simulink library "Condensing_Boiler_CONF"  (R2013b)
settings: Solver=ode45  StartTime=0.0  StopTime=10.0  RelTol=1e-3
libraries: carnot x1
settings Model: Creator=lena.frank  LastModifiedBy=drhf

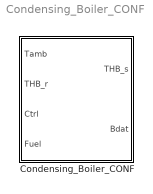
== system Condensing_Boiler_CONF ==
  Condensing_Boiler_CONF : Subsystem  mask(Configurated Condensing Boiler){parameterfile=DefaultCondensingBoiler, tini=20}
      mask prompts: parameterfile "Parameter set"; tini "Inital temperature in °C"
      mask help:
      | Multinode one-dimensional model of a boiler. Condensing effects are taken in account by an efficiency lookup table.
      | This block uses predefined parameter sets.
      mask init:
      | B = CarnotCallbacks_CondensingBoilerConf(parameterfile);
      | relQdotMin = B.QdotMin/B.Qdotnom;
      mask Help: web(fullfile(path_carnot('help'),'Condensing_Boiler_CONF.html'),'-helpbrowser')
      mask TypeOptions parameterfile: DefaultCondensingBoiler | Vitodens_200_13kW | Vitodens_200_19kW | Vitodens_200_26kW | Vitodens_200_35kW
      mask Display:
      | % user defined picture file
      | picfile = fullfile(path_carnot('intlibsl'), ...
      |         'Source','Boiler','Condensing_Boiler_CONF','parameter_set', ...
      |         'Condensing_Boiler_CONF.jpg');
      | 
      | pic = false;
      | if ~BlockIsInCarnotLibrary    % if not located in library any more
      |     if exist(picfile,'file') % show internal picture if defined
      |         image(imread(picfile), [0.2, 0, 0.6, 1])
      |         set_param(gcb, 'BackgroundColor', 'White')
      |         pic = true;
      |     end
      | end
      | if ~pic    % show public picture
      |     set_param(gcb, 'BackgroundColor', 'Red')
      |     plot(0,0,1,1,[10,90,90,10,10]/100,[10,10,20,20,10]/100,[80,80,20,20]/100, ...
      |         [20,90,90,20]/100,[20,70,70,20]/100,[24,24,30,30]/100,[32,30,28]/100, ...
      |         [30,40,30]/100,[43,40,38]/100,[30,40,30]/100,[53,50,47]/100, ...
      |         [30,40,30]/100,[63,60,57]/100,[30,40,30]/100, ...
      |         [35,32,30,29,31,36,39,40,37,35]/100,[75,69,65,58,50,49,53,59,68,75]/100, ...
      |         [57,54,51,51,53,58,62,62,59,57]/100,[76,71,67,58,49,48,54,60,69,76]/100)
      | end
      | 
      | % Show port labels: same as port labels in the subsystem,
      | % but display with a picture covers the text. Have to reprint it.
      | port_label('input',1,'Tamb')
      | port_label('input',2,'THB_r')
      | port_label('input',3,'Ctrl')
      | port_label('input',4,'Fuel')
      | port_label('output',1,'THB_s')
      | port_label('output',2,'Bdat')

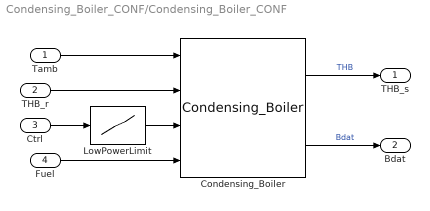
== system Condensing_Boiler_CONF/Condensing_Boiler_CONF ==
  Tamb : Inport
  THB_r : Inport  Port=2
  Ctrl : Inport  Port=3
  Fuel : Inport  Port=4
  Condensing_Boiler : carnot/Source/Boiler/Condensing_Boiler  Pnom=B.Qdotnom  U=B.HeatLoss  vol=B.Volume  electricPower=B.ElectricPower  relativeQdot=B.TableRelativePower  whichTforEfficiency=mean of inlet and outlet temperature  temperatures=B.TableTemperatures  efficiency=B.TableData  lin=B.dplin  qua=B.dpqua  Tini=tini  nodes=B.Nodes
  LowPowerLimit : Lookup  InputValues=[-1, relQdotMin-eps, relQdotMin, 1, 2]  Table=[0, 0, relQdotMin, 1, 1]
  THB_s : Outport
  Bdat : Outport  Port=2
  wires:
  Fuel/1 -> Condensing_Boiler/4
  Condensing_Boiler/2 -> Bdat/1  "Bdat"
  Condensing_Boiler/1 -> THB_s/1  "THB"
  Tamb/1 -> Condensing_Boiler/1
  Ctrl/1 -> LowPowerLimit/1
  THB_r/1 -> Condensing_Boiler/2
  LowPowerLimit/1 -> Condensing_Boiler/3
